simulink model "BicycleMDL_sine"  (R2016b)
settings: Solver=ode1  StartTime=0.0  StopTime=10.0  FixedStep=dt  RelTol=1e-3
values from neighbouring files (symbols this model uses):
  A = [(-(a^2)*c_f-(b^2)*c_r)/(I*v_x) (-(a)*c_f+(b)*c_r)/I 0 0; (-(a)*c_f+(b)*c_r-m*(v_x)^2)/(m*(v_x)^2),(-c_f-c_r)/(m*(v_x)) 0 0;     1,0,0,0 ... (first row only)    [Bycicle_Model_2_old.m]    (also in Run_model.m = [(-((a^2)*c_f+(b^2)*c_r))/(I_z*v_x) (-(a)*c_f+(b)*c_r)/(I_z*)
  B = [a*c_f/I,0;     c_f/(m*c_f),0;     0,-v_x ... (first row only)    [Bycicle_Model_2_old.m]    (also in Run_model.m = [a*c_f/I_z,0;     c_f/(m),0;     0,v_x)
  C = [1,0,0,0;     (-(a)*c_f+(b)*c_r)/(m*v_x),(-c_f-c_r+m*a_x)/m,0,0;     0,0,1,0;     0,0,0,1]    [Bycicle_Model_2_old.m]    (also in Run_model.m = [1,0,0,0;     0,1,0,0;     0,0,1,0;     0,0,0,1;     0,1/v_x)
  D = [0,0;     c_f/(m),0;     0,0 ... (first row only)    [Bycicle_Model_2_old.m]    (also in Run_model.m = [0 0; 0 0; 0 0; 0 0; 0 0; 0 0])
  dt = 0.001    [Run_model.m]
settings Model: Creator=rwouters  LastModifiedBy=rwouters

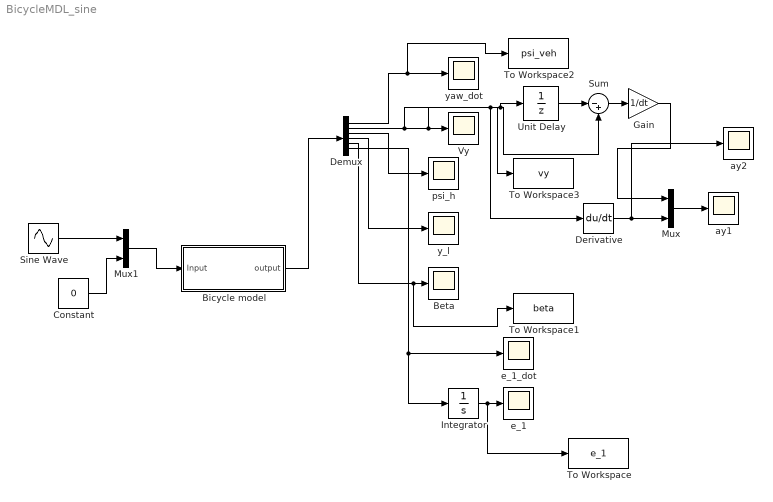
== system BicycleMDL_sine ==
  Beta : Scope
  Bicycle model : Subsystem
  Constant : Constant  Value=0
  Demux : Demux  Outputs=6
  Derivative : Derivative
  Gain : Gain  Gain=1/dt
  Integrator : Integrator
  Mux : Mux  Inputs=2
  Mux1 : Mux  Inputs=2
  Sine Wave : Sin  Amplitude=0.01  Frequency=3  SampleTime=0
  Sum : Sum  Inputs=|-+
  To Workspace : ToWorkspace  VariableName=e_1  SaveFormat=Timeseries  SampleTime=-1
  To Workspace1 : ToWorkspace  VariableName=beta  SaveFormat=Timeseries  SampleTime=-1
  To Workspace2 : ToWorkspace  VariableName=psi_veh  SaveFormat=Timeseries  SampleTime=-1
  To Workspace3 : ToWorkspace  VariableName=vy  SaveFormat=Timeseries  SampleTime=-1
  Unit Delay : UnitDelay  SampleTime=-1
  Vy : Scope
  ay1 : Scope
  ay2 : Scope
  e_1 : Scope
  e_1_dot : Scope
  psi_h : Scope
  y_l : Scope
  yaw_dot : Scope
  wires:
  Bicycle model/1(output) -> Demux/1
  Demux/1 -> To Workspace2/1, yaw_dot/1
  Demux/3 -> psi_h/1
  Demux/4 -> y_l/1
  Demux/5 -> To Workspace1/1, Beta/1
  Demux/6 -> Integrator/1, e_1_dot/1
  Integrator/1 -> To Workspace/1, e_1/1
  Demux/2 -> Vy/1, Sum/2, Unit Delay/1, Derivative/1, To Workspace3/1
  Gain/1 -> Mux/1
  Unit Delay/1 -> Sum/1
  Sum/1 -> Gain/1
  Derivative/1 -> ay2/1, Mux/2
  Mux/1 -> ay1/1
  Mux1/1 -> Bicycle model/1(Input)
  Constant/1 -> Mux1/2
  Sine Wave/1 -> Mux1/1

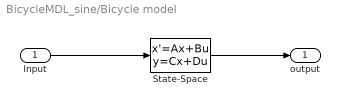
== system BicycleMDL_sine/Bicycle model ==
  Input : Inport
  State-Space : StateSpace  A=A  B=B  C=C  D=D  X0=[0 0 0 0]
  output : Outport
  wires:
  Input/1 -> State-Space/1
  State-Space/1 -> output/1
